simulink model "ambasMalhas"  (R2022b)
settings: Solver=VariableStepAuto  StartTime=0.0  StopTime=30  RelTol=1e-3
values from neighbouring files (symbols this model uses):
  Cd = ss_d.C    [lab6.m]
  Dd = ss_d.D    [lab6.m]
  disturbio = 0.24    [lab6.m]
  F = ss_d.A    [lab6.m]
  H = ss_d.B    [lab6.m]
  R = 1.18    [lab6.m]
  T0 = 1/F0    [lab6.m]
undefined symbols (not defined in the file or in its folder): Ac, Bc, Cc, Dc
settings Model: Creator=mathe  LastModifiedBy=mathe

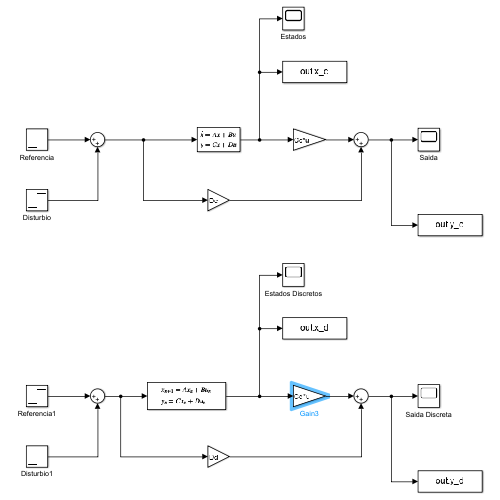
[thumbnail: Simulink's stored preview of the top-level diagram]
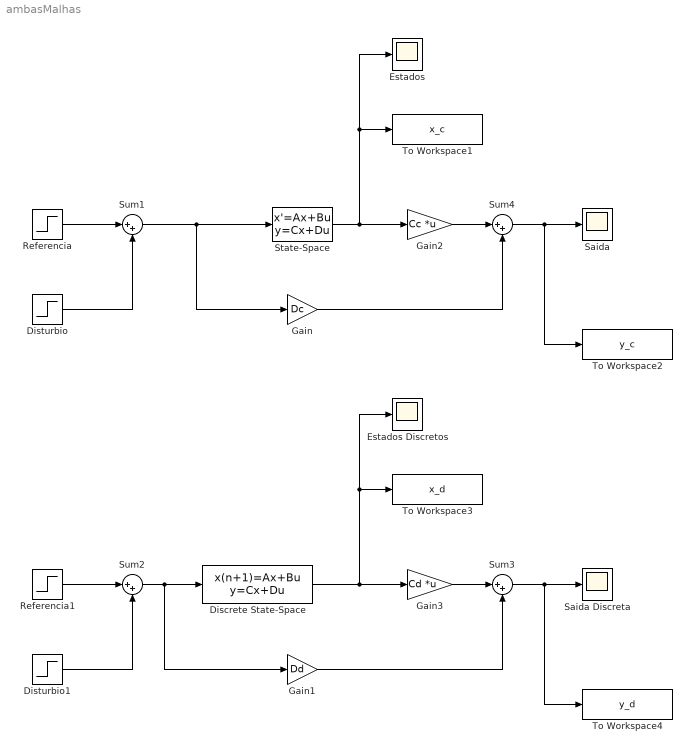
== system ambasMalhas ==
  Discrete State-Space : DiscreteStateSpace  A=F  B=H  C=[1 0;0 1]  D=[0;0]  SampleTime=T0
  Disturbio : Step  Time=15  After=disturbio  SampleTime=0
  Disturbio1 : Step  Time=15  After=disturbio  SampleTime=0
  Estados : Scope
  Estados Discretos : Scope
  Gain : Gain  Gain=Dc
  Gain1 : Gain  Gain=Dd
  Gain2 : Gain  Gain=Cc  Multiplication=Matrix(K*u)
  Gain3 : Gain  Gain=Cd  Multiplication=Matrix(K*u)
  Referencia : Step  Time=0  After=R  SampleTime=0
  Referencia1 : Step  Time=0  After=R  SampleTime=0
  Saida : Scope
  Saida Discreta : Scope
  State-Space : StateSpace  A=Ac  B=Bc  C=[1 0; 0 1]  D=[0; 0]  InitialCondition=0
  Sum{1..4} (4 alike) : Sum  Inputs=|++
  To Workspace1 : ToWorkspace  VariableName=x_c  SaveFormat=Timeseries  SampleTime=-1
  To Workspace2 : ToWorkspace  VariableName=y_c  SaveFormat=Timeseries  SampleTime=-1
  To Workspace3 : ToWorkspace  VariableName=x_d  SaveFormat=Timeseries  SampleTime=-1
  To Workspace4 : ToWorkspace  VariableName=y_d  SaveFormat=Timeseries  SampleTime=-1
  wires:
  State-Space/1 -> Gain2/1, Estados/1, To Workspace1/1
  Sum4/1 -> To Workspace2/1, Saida/1
  Sum1/1 -> State-Space/1, Gain/1
  Referencia/1 -> Sum1/1
  Disturbio/1 -> Sum1/2
  Gain2/1 -> Sum4/1
  Gain/1 -> Sum4/2
  Discrete State-Space/1 -> Gain3/1, Estados Discretos/1, To Workspace3/1
  Sum3/1 -> To Workspace4/1, Saida Discreta/1
  Gain1/1 -> Sum3/2
  Referencia1/1 -> Sum2/1
  Gain3/1 -> Sum3/1
  Disturbio1/1 -> Sum2/2
  Sum2/1 -> Discrete State-Space/1, Gain1/1
